simulink model "System Modelling"  (R2015b)
settings: Solver=VariableStepAuto  StartTime=0.0  StopTime=10.0  RelTol=1e-3
settings Model: Creator=acer  LastModifiedBy=acer

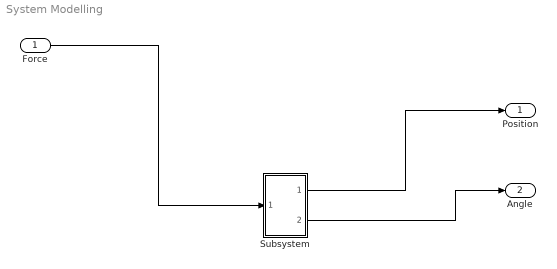
== system System Modelling ==
  Force : Inport
  Subsystem : Subsystem
  Position : Outport
  Angle : Outport  Port=2
  wires:
  Force/1 -> Subsystem/1(Force)
  Subsystem/1(Position) -> Position/1
  Subsystem/2(Angle) -> Angle/1

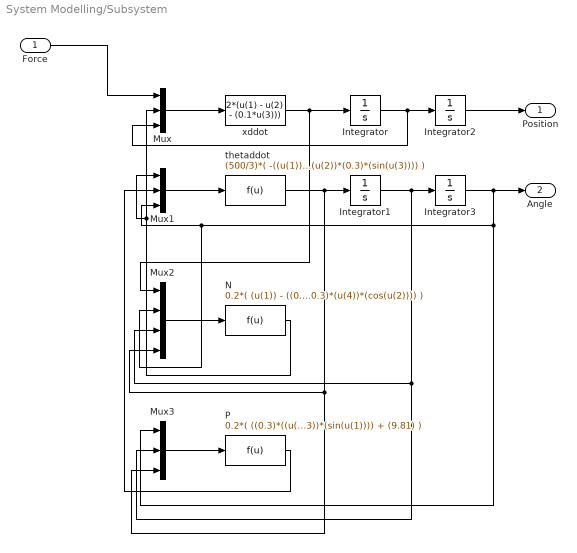
== system System Modelling/Subsystem ==
  Force : Inport
  Integrator : Integrator  ContinuousStateAttributes='xdot'
  Integrator1 : Integrator  ContinuousStateAttributes='thetadot'
  Integrator2 : Integrator  InitialCondition=pi  ContinuousStateAttributes='x'
  Integrator3 : Integrator  InitialCondition=pi  ContinuousStateAttributes='theta'
  Mux : Mux  Inputs=3
  Mux1 : Mux  Inputs=3
  Mux2 : Mux
  Mux3 : Mux  Inputs=3
  N : Fcn  Expr=0.2*( (u(1)) - ((0.3)*((u(3))^2)*(sin(u(2)))) + ((0.3)*(u(4))*(cos(u(2)))) )
  P : Fcn  Expr=0.2*( ((0.3)*((u(2))^2)*(cos(u(1)))) + ((0.3)*(u(3))*(sin(u(1)))) + (9.81) )
  thetaddot : Fcn  Expr=(500/3)*( -((u(1))*(0.3)*(cos(u(3)))) - ((u(2))*(0.3)*(sin(u(3)))) )
  xddot : Fcn  Expr=2*(u(1) - u(2) - (0.1*u(3)))
  Position : Outport
  Angle : Outport  Port=2
  wires:
  thetaddot/1 -> Mux3/3, Mux2/4, Integrator1/1
  N/1 -> Mux1/1, Mux/2
  P/1 -> Mux1/2
  Integrator/1 -> Mux/3, Integrator2/1
  xddot/1 -> Mux2/1, Integrator/1
  Mux3/1 -> P/1
  Integrator1/1 -> Mux3/2, Mux2/3, Integrator3/1
  Force/1 -> Mux/1
  Integrator3/1 -> Angle/1, Mux3/1, Mux2/2, Mux1/3
  Integrator2/1 -> Position/1
  Mux/1 -> xddot/1
  Mux1/1 -> thetaddot/1
  Mux2/1 -> N/1
